simulink model "FOC"  (Simulink 7.5)
settings: Solver=ode3  StartTime=0.0  StopTime=1  FixedStep=1e-5  RelTol=1e-3
libraries: powerlib x5, simulink x1
settings Model: Creator=lenovo  LastModifiedBy=Administrator

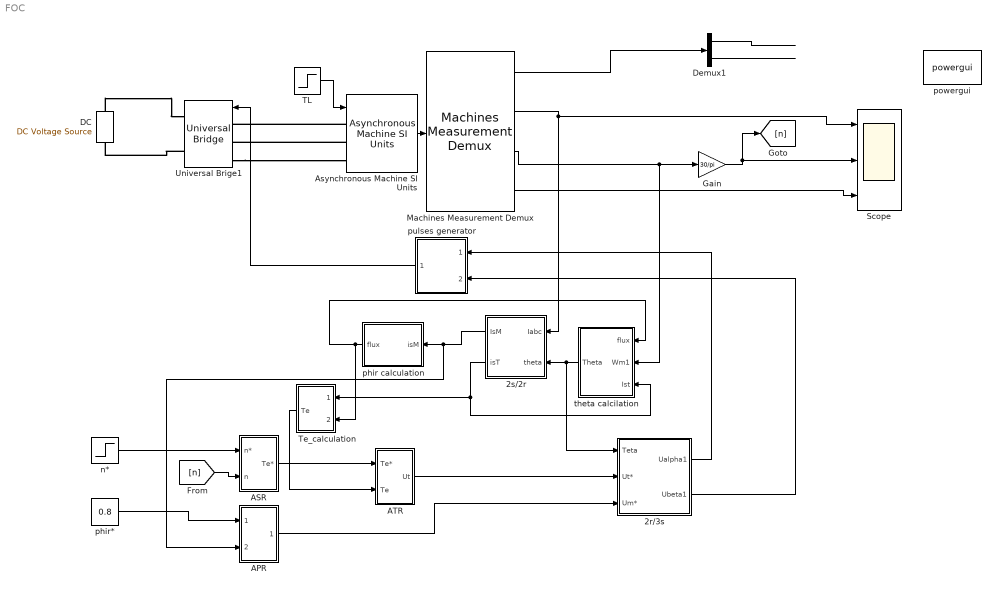
== system FOC ==
  2r/3s : Subsystem
  2s/2r : Subsystem
  APR : Subsystem
  ASR : Subsystem
  ATR : Subsystem
  Asynchronous Machine SI Units : powerlib/Machines/Asynchronous Machine SI Units  DialogController=POWERSYS.PowerSysDialog  SystemSampleTime=-1  PresetModel="17:  20 HP (15KW)   400 V 50Hz 1460 RPM"  MechanicalLoad=Torque Tm  ShowDetailedParameters=on  RotorType=Squirrel-cage  ReferenceFrame=Stationary  NominalParameters=[1.5e+004 400 50]  Stator=[0.2147 0.000991]  Rotor=[0.2205 0.000991]  Lm=0.06419  Mechanical=[0.102 0.009541 2]  PolePairs=2  InitialConditions="[ 1,0   0,0,0   0,0,0 ]"  Units=SI  LoadFlowParameters=0  SimulateSaturation=off  Saturation=[9.9249,19.6672,38.0377,51.3988,69.2824,105.1337,152.5532,214.2421,303.1917;230, 322, 414, 460, 506, 552, 598, 644, 690]  TsPowergui=0  TsBlock=-1  IterativeModel=Forward Euler
  "DC " : powerlib/Electrical Sources/DC Voltage Source  DialogController=POWERSYS.PowerSysDialog  SystemSampleTime=-1  Amplitude=650  Measurements=None
  Demux1 : Demux  Outputs=2
  Gain : Gain  Gain=30/pi
  Machines Measurement Demux : powerlib/Machines/Machines Measurement Demux  DialogController=POWERSYS.PowerSysDialog  SystemSampleTime=-1  machType=Asynchronous  ssm1=on  ssm2=on  ssm3=on  ssm4=on  ssm5=on  ssm6=on  sm1=off  sm2=off  sm3=off  sm4=off  sm5=off  sm6=off  sm7=off  sm8=on  sm9=off  sm10=off  sm11=off  sm115=off  sm12=off  sm13=off  sm14=off  asm1=off  asm2=off  asm3=on  asm4=off  asm5=on  asm6=off  asm7=off  asm8=off  asm9=on  asm10=on  asm11=off  pmsm1=on  pmsm2=on  pmsm3=on  pmsm4=off  pmsm5=on  pmsm6=on  pmsm7=on  lastType=1
  Scope : Scope  NumInputPorts=3
      settings: YMin=-400~0~-250  YMax=450~1500~350  SaveName=ScopeData3
  TL : Step  Time=0.4  After=0  SampleTime=0
  Te_calculation : Subsystem
  Universal Brige1 : powerlib/Power Electronics/Universal Bridge  DialogController=POWERSYS.PowerSysDialog  SystemSampleTime=-1  Arms=3  SnubberResistance=1e5  SnubberCapacitance=inf  Device=IGBT / Diodes  Ron=1e-3  Lon=0  ForwardVoltages="[  0  0  ]"  ForwardVoltage=0  GTOparameters=[ 10e-6 , 20e-6 ]  IGBTparameters=[ 1e-6 , 2e-6 ]  Measurements=All voltages and currents  Measurements_2=None  converterType=Rectifier
  n* : Step  Time=0.5  Before=1420  After=1200  SampleTime=0
  phir calculation : Subsystem
  phir* : Constant  Value=0.8
  powergui : powerlib/powergui  Priority=1  SystemSampleTime=-1  SimulationMode=Continuous  SampleTime=50e-6  frequency=60  SPID=off  DisableSnubberDevices=off  DisableRonSwitches=off  DisableVfSwitches=off  SwTol=0  Interpol=off  frequencyindice=50  echomessages=off  HookPort=off  DisplayEquations=off  FunctionMessages=off  EnableUseOfTLC=off  x0status=blocks  RestoreLinks=warning  ResistiveCurrentMeasurement=off  Ylog=off  Xlog=on  ShowGrid=off  save=off  variable=ZData  ZoomFFT=off  StartTime=0.0  cycles=1  DisplayStyle=1  FreqAxis=off  MaxFrequency=1000  frequencyindicesteady=1  display=off  methode=off
  pulses generator : Subsystem
  theta calcilation : Subsystem
  wires:
  TL/1 -> Asynchronous Machine SI Units/1
  phir calculation/1(flux) -> Te_calculation/2(flux), theta calcilation/1(flux)
  n*/1 -> ASR/1(n*)
  ATR/1(Ut) -> 2r/3s/2(Ut*)
  phir*/1 -> APR/1(phir*)
  APR/1(Um) -> 2r/3s/3(Um*)
  Asynchronous Machine SI Units/1 -> Machines Measurement Demux/1
  Machines Measurement Demux/2 -> Scope/1, 2s/2r/1(Iabc)
  Machines Measurement Demux/3 -> Gain/1, theta calcilation/2(Wm1)
  Gain/1 -> [n], Scope/2
  [n] -> ASR/2(n)
  Machines Measurement Demux/4 -> Scope/3
  2s/2r/1(IsM) -> phir calculation/1(isM), APR/2(phir)
  theta calcilation/1(Theta) -> 2s/2r/2(theta), 2r/3s/1(Teta)
  2s/2r/2(isT) -> theta calcilation/3(Ist), Te_calculation/1(i_sT)
  Machines Measurement Demux/1 -> Demux1/1
  ASR/1(Te*) -> ATR/1(Te*)
  pulses generator/1(SVPWM) -> Universal Brige1/1
  2r/3s/1(Ualpha1) -> pulses generator/1(Ualpha)
  2r/3s/2(Ubeta1) -> pulses generator/2(Ubeta)
  Demux1/1 -> ?
  Demux1/2 -> ?
  Te_calculation/1(Te) -> ATR/2(Te)
  connections:
  "DC "/RConn1 -- Universal Brige1/RConn1
  Universal Brige1/RConn2 -- "DC "/LConn1
  Asynchronous Machine SI Units/LConn1 -- Universal Brige1/LConn1
  Asynchronous Machine SI Units/LConn2 -- Universal Brige1/LConn2
  Universal Brige1/LConn3 -- Asynchronous Machine SI Units/LConn3

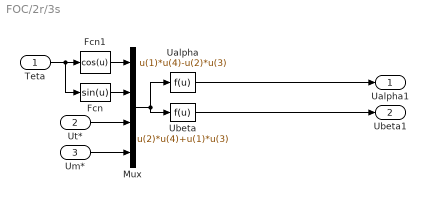
== system FOC/2r/3s ==
  Teta : Inport
  Ut* : Inport  Port=2
  Um* : Inport  Port=3
  Fcn : Fcn  Expr=sin(u)
  Fcn1 : Fcn  Expr=cos(u)
  Mux : Mux
  Ualpha : Fcn  Expr=u(1)*u(4)-u(2)*u(3)
  Ubeta : Fcn  Expr=u(2)*u(4)+u(1)*u(3)
  Ualpha1 : Outport  InitialOutput=0
  Ubeta1 : Outport  Port=2  InitialOutput=0
  wires:
  Um*/1 -> Mux/4
  Ut*/1 -> Mux/3
  Teta/1 -> Fcn/1, Fcn1/1
  Mux/1 -> Ualpha/1, Ubeta/1
  Fcn1/1 -> Mux/1
  Fcn/1 -> Mux/2
  Ualpha/1 -> Ualpha1/1
  Ubeta/1 -> Ubeta1/1

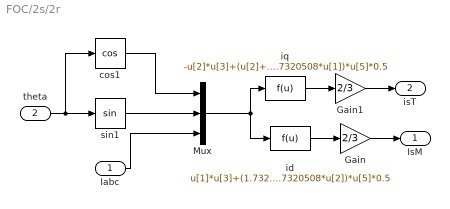
== system FOC/2s/2r ==
  Iabc : Inport
  theta : Inport  Port=2
  Gain : Gain  Gain=2/3  SaturateOnIntegerOverflow=on  OutDataTypeStr=Inherit: Same as input  ParamDataTypeStr=Inherit: Same as input
  Gain1 : Gain  Gain=2/3  SaturateOnIntegerOverflow=on  OutDataTypeStr=Inherit: Same as input  ParamDataTypeStr=Inherit: Same as input
  Mux : Mux  Inputs=3
  cos1 : Trigonometry  Operator=cos
  id : Fcn  Expr=u[1]*u[3]+(1.7320508*u[2]-u[1])*u[4]*0.5+(-u[1]-1.7320508*u[2])*u[5]*0.5
  iq : Fcn  Expr=-u[2]*u[3]+(u[2]+1.7320508*u[1])*u[4]*0.5+(u[2]-1.7320508*u[1])*u[5]*0.5
  sin1 : Trigonometry
  IsM : Outport  InitialOutput=0
  isT : Outport  Port=2  InitialOutput=0
  wires:
  Iabc/1 -> Mux/3
  iq/1 -> Gain1/1
  id/1 -> Gain/1
  Gain/1 -> IsM/1
  Gain1/1 -> isT/1
  Mux/1 -> iq/1, id/1
  cos1/1 -> Mux/1
  sin1/1 -> Mux/2
  theta/1 -> sin1/1, cos1/1

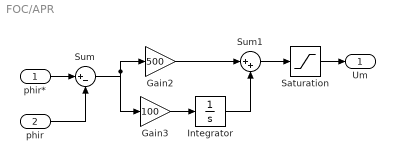
== system FOC/APR ==
  phir* : Inport
  phir : Inport  Port=2
  Gain2 : Gain  Gain=500
  Gain3 : Gain  Gain=100
  Integrator : Integrator  LimitOutput=on  UpperSaturationLimit=13  LowerSaturationLimit=-13
  Saturation : Saturate  UpperLimit=500  LowerLimit=-500
  Sum : Sum  Inputs=|+-
  Sum1 : Sum  Inputs=|++
  Um : Outport
  wires:
  Sum/1 -> Gain2/1, Gain3/1
  Gain2/1 -> Sum1/1
  Gain3/1 -> Integrator/1
  Integrator/1 -> Sum1/2
  Sum1/1 -> Saturation/1
  Saturation/1 -> Um/1
  phir*/1 -> Sum/1
  phir/1 -> Sum/2

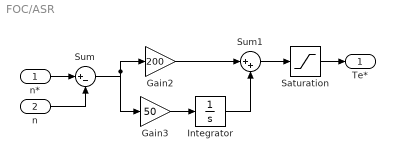
== system FOC/ASR ==
  n* : Inport
  n : Inport  Port=2
  Gain2 : Gain  Gain=200
  Gain3 : Gain  Gain=50
  Integrator : Integrator  LimitOutput=on  UpperSaturationLimit=200  LowerSaturationLimit=-200
  Saturation : Saturate  UpperLimit=200  LowerLimit=-200
  Sum : Sum  Inputs=|+-
  Sum1 : Sum  Inputs=|++
  Te* : Outport
  wires:
  Sum/1 -> Gain2/1, Gain3/1
  Gain2/1 -> Sum1/1
  Gain3/1 -> Integrator/1
  Integrator/1 -> Sum1/2
  Sum1/1 -> Saturation/1
  Saturation/1 -> Te*/1
  n*/1 -> Sum/1
  n/1 -> Sum/2

== system FOC/ATR ==
  Te* : Inport
  Te : Inport  Port=2
  Gain2 : Gain  Gain=500
  Gain3 : Gain  Gain=50
  Integrator : Integrator  LimitOutput=on  UpperSaturationLimit=200  LowerSaturationLimit=-80
  Saturation : Saturate  UpperLimit=500  LowerLimit=-500
  Sum : Sum  Inputs=|+-
  Sum1 : Sum  Inputs=|++
  Ut : Outport
  wires:
  Sum/1 -> Gain2/1, Gain3/1
  Gain2/1 -> Sum1/1
  Gain3/1 -> Integrator/1
  Integrator/1 -> Sum1/2
  Sum1/1 -> Saturation/1
  Saturation/1 -> Ut/1
  Te*/1 -> Sum/1
  Te/1 -> Sum/2

== system FOC/Te_calculation ==
  i_sT : Inport  OutDataType=fixdt(1, 16)  OutScaling=2^0
  flux : Inport  Port=2  OutDataType=fixdt(1, 16)  OutScaling=2^0
  Gain : Gain  Gain=1/0.50771927  ParameterDataType=fixdt(1, 16)  ParameterScaling=2^0  OutDataType=fixdt(1, 16)  OutScaling=2^0
  Product : Product  OutDataType=fixdt(1, 16)  OutScaling=2^0  RndMeth=Zero
  Te : Outport  OutDataType=fixdt(1, 16)  OutScaling=2^0
  wires:
  flux/1 -> Product/2
  i_sT/1 -> Gain/1
  Product/1 -> Te/1
  Gain/1 -> Product/1

== system FOC/phir calculation ==
  isM : Inport
  Transfer Fcn : TransferFcn  Numerator=[0.06419]  Denominator=[0.2956 1]
  flux : Outport
  wires:
  isM/1 -> Transfer Fcn/1
  Transfer Fcn/1 -> flux/1

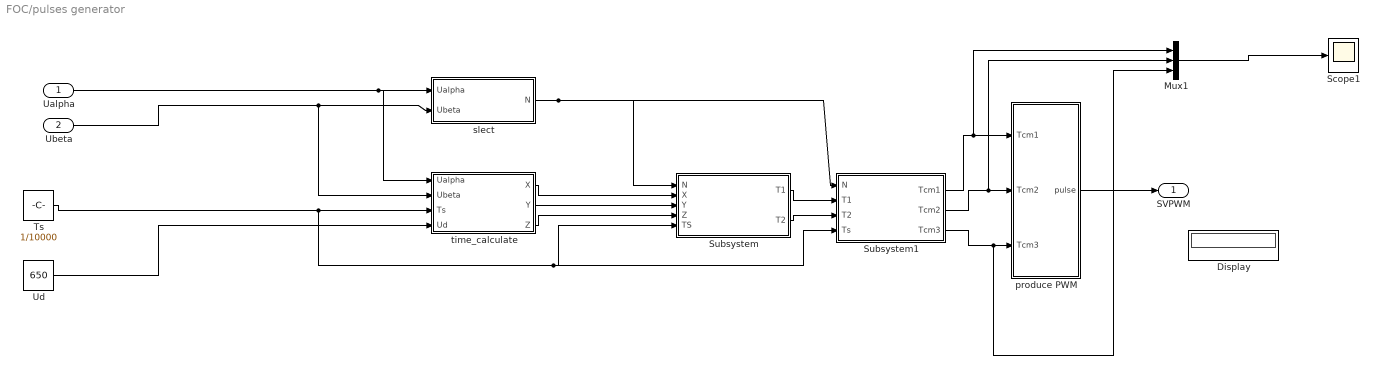
== system FOC/pulses generator ==
  Ualpha : Inport  OutDataType=fixdt(1, 16)  OutScaling=2^0
  Ubeta : Inport  Port=2  OutDataType=fixdt(1, 16)  OutScaling=2^0
  Display : Display
  Mux1 : Mux  Inputs=3
  Scope1 : Scope
      settings: TimeRange=0.2  YMin=3.5e-005  YMax=6.5e-005  SaveName=ScopeData2
  Subsystem : Subsystem
  Subsystem1 : Subsystem
  Ts : Constant  Value=1/10000  OutDataType=fixdt(1, 16)  OutScaling=2^0
  Ud : Constant  Value=650  OutDataType=fixdt(1, 16)  OutScaling=2^0
  produce PWM : Subsystem
  slect : Subsystem
  time_calculate : Subsystem
  SVPWM : Outport  OutDataType=fixdt(1, 16)  OutScaling=2^0
  wires:
  Ualpha/1 -> time_calculate/1(Ualpha), slect/1(Ualpha)
  slect/1(N) -> Subsystem/1(N), Subsystem1/1(N)
  Subsystem/1(T1) -> Subsystem1/2(T1)
  Subsystem/2(T2) -> Subsystem1/3(T2)
  Subsystem1/1(Tcm1) -> produce PWM/1(Tcm1), Mux1/1
  Ts/1 -> time_calculate/3(Ts), Subsystem/5(TS), Subsystem1/4(Ts)
  Ud/1 -> time_calculate/4(Ud)
  Subsystem1/2(Tcm2) -> produce PWM/2(Tcm2), Mux1/2
  Subsystem1/3(Tcm3) -> produce PWM/3(Tcm3), Mux1/3
  time_calculate/1(X) -> Subsystem/2(X)
  time_calculate/2(Y) -> Subsystem/3(Y)
  time_calculate/3(Z) -> Subsystem/4(Z)
  Mux1/1 -> Scope1/1
  Ubeta/1 -> slect/2(Ubeta), time_calculate/2(Ubeta)
  produce PWM/1(pulse) -> SVPWM/1

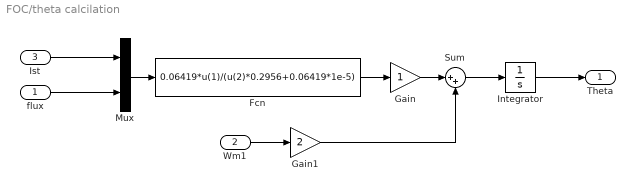
== system FOC/theta calcilation ==
  flux : Inport
  Wm1 : Inport  Port=2
  Ist : Inport  Port=3
  Fcn : Fcn  Expr=0.06419*u(1)/(u(2)*0.2956+0.06419*1e-5)
  Gain : Gain
  Gain1 : Gain  Gain=2
  Integrator : Integrator  InitialCondition=1e-6  LimitOutput=on  UpperSaturationLimit=1e6  LowerSaturationLimit=-1e6
  Mux : Mux  Inputs=2
  Sum : Sum  Inputs=|++
  Theta : Outport
  wires:
  Ist/1 -> Mux/1
  flux/1 -> Mux/2
  Mux/1 -> Fcn/1
  Fcn/1 -> Gain/1
  Gain/1 -> Sum/1
  Gain1/1 -> Sum/2
  Sum/1 -> Integrator/1
  Integrator/1 -> Theta/1
  Wm1/1 -> Gain1/1

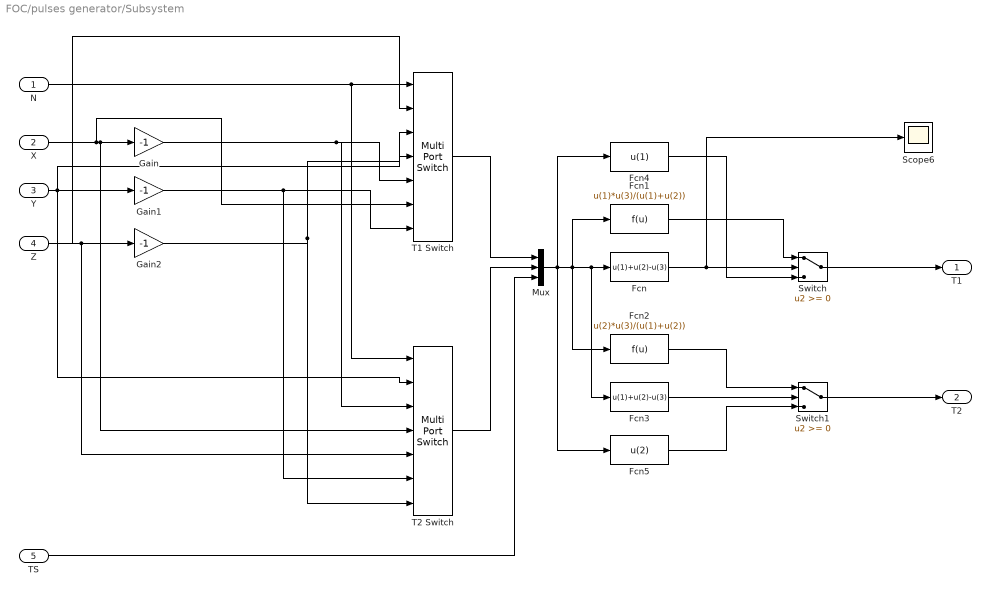
== system FOC/pulses generator/Subsystem ==
  N : Inport  OutDataType=fixdt(1, 16)  OutScaling=2^0
  X : Inport  Port=2  OutDataType=fixdt(1, 16)  OutScaling=2^0
  Y : Inport  Port=3  OutDataType=fixdt(1, 16)  OutScaling=2^0
  Z : Inport  Port=4  OutDataType=fixdt(1, 16)  OutScaling=2^0
  TS : Inport  Port=5  OutDataType=fixdt(1, 16)  OutScaling=2^0
  Fcn : Fcn  Expr=u(1)+u(2)-u(3)
  Fcn1 : Fcn  Expr=u(1)*u(3)/(u(1)+u(2))
  Fcn2 : Fcn  Expr=u(2)*u(3)/(u(1)+u(2))
  Fcn3 : Fcn  Expr=u(1)+u(2)-u(3)
  Fcn4 : Fcn  Expr=u(1)
  Fcn5 : Fcn  Expr=u(2)
  Gain : Gain  Gain=-1  ParameterDataType=fixdt(1, 16)  ParameterScaling=2^0  OutDataType=fixdt(1, 16)  OutScaling=2^0
  Gain1 : Gain  Gain=-1  ParameterDataType=fixdt(1, 16)  ParameterScaling=2^0  OutDataType=fixdt(1, 16)  OutScaling=2^0
  Gain2 : Gain  Gain=-1  ParameterDataType=fixdt(1, 16)  ParameterScaling=2^0  OutDataType=fixdt(1, 16)  OutScaling=2^0
  Mux : Mux  Inputs=3
  Scope6 : Scope
      settings: TimeRange=0.2  YMin=-1.05e-005  YMax=-4e-006  SaveName=ScopeData5  SampleTime=0.000001
  Switch : Switch  OutDataType=fixdt(1, 16)  OutScaling=2^0
  Switch1 : Switch  OutDataType=fixdt(1, 16)  OutScaling=2^0
  T1 Switch : MultiPortSwitch  Inputs=6  zeroidx=off  OutDataType=fixdt(1, 16)  OutScaling=2^0
  T2 Switch : MultiPortSwitch  Inputs=6  zeroidx=off  OutDataType=fixdt(1, 16)  OutScaling=2^0
  T1 : Outport  OutDataType=fixdt(1, 16)  OutScaling=2^0
  T2 : Outport  Port=2  OutDataType=fixdt(1, 16)  OutScaling=2^0
  wires:
  N/1 -> T1 Switch/1, T2 Switch/1
  X/1 -> Gain/1, T2 Switch/4, T1 Switch/6
  Y/1 -> Gain1/1, T2 Switch/2, T1 Switch/3
  Z/1 -> Gain2/1, T1 Switch/2, T2 Switch/5
  Gain/1 -> T2 Switch/3, T1 Switch/5
  Gain2/1 -> T1 Switch/4, T2 Switch/7
  Gain1/1 -> T2 Switch/6, T1 Switch/7
  T1 Switch/1 -> Mux/1
  T2 Switch/1 -> Mux/2
  TS/1 -> Mux/3
  Mux/1 -> Fcn1/1, Fcn/1, Fcn3/1, Fcn2/1, Fcn4/1, Fcn5/1
  Fcn3/1 -> Switch1/2
  Switch/1 -> T1/1
  Switch1/1 -> T2/1
  Fcn4/1 -> Switch/3
  Fcn/1 -> Switch/2, Scope6/1
  Fcn1/1 -> Switch/1
  Fcn2/1 -> Switch1/1
  Fcn5/1 -> Switch1/3

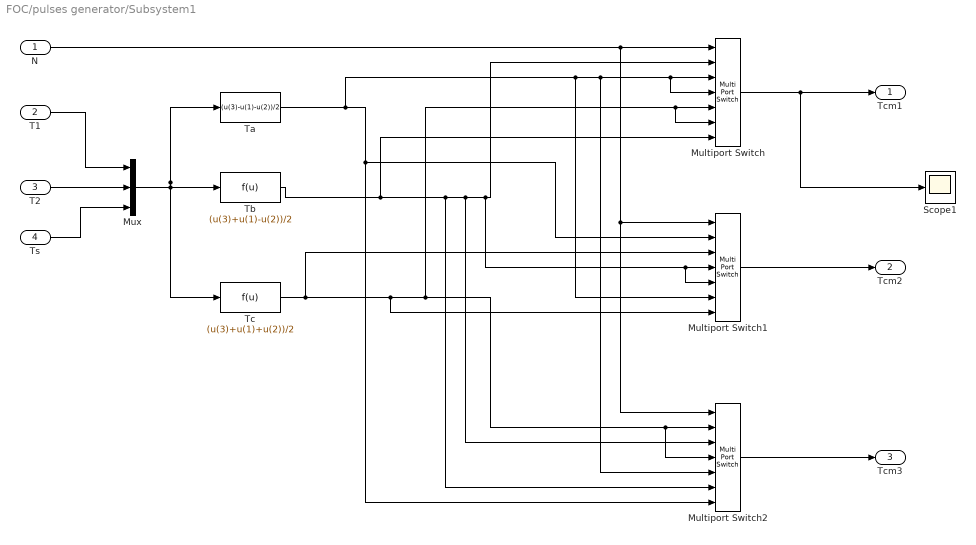
== system FOC/pulses generator/Subsystem1 ==
  N : Inport  OutDataType=fixdt(1, 16)  OutScaling=2^0
  T1 : Inport  Port=2  OutDataType=fixdt(1, 16)  OutScaling=2^0
  T2 : Inport  Port=3  OutDataType=fixdt(1, 16)  OutScaling=2^0
  Ts : Inport  Port=4  OutDataType=fixdt(1, 16)  OutScaling=2^0
  Multiport Switch : MultiPortSwitch  Inputs=6  zeroidx=off  OutDataType=fixdt(1, 16)  OutScaling=2^0
  Multiport Switch1 : MultiPortSwitch  Inputs=6  zeroidx=off  OutDataType=fixdt(1, 16)  OutScaling=2^0
  Multiport Switch2 : MultiPortSwitch  Inputs=6  zeroidx=off  OutDataType=fixdt(1, 16)  OutScaling=2^0
  Mux : Mux  Inputs=3
  Scope1 : Scope
      settings: YMin=-2.5e-006  YMax=2.75e-005  SaveName=ScopeData4
  Ta : Fcn  Expr=(u(3)-u(1)-u(2))/2
  Tb : Fcn  Expr=(u(3)+u(1)-u(2))/2
  Tc : Fcn  Expr=(u(3)+u(1)+u(2))/2
  Tcm1 : Outport  OutDataType=fixdt(1, 16)  OutScaling=2^0
  Tcm2 : Outport  Port=2  OutDataType=fixdt(1, 16)  OutScaling=2^0
  Tcm3 : Outport  Port=3  OutDataType=fixdt(1, 16)  OutScaling=2^0
  wires:
  Ts/1 -> Mux/3
  Multiport Switch/1 -> Tcm1/1, Scope1/1
  Multiport Switch1/1 -> Tcm2/1
  Multiport Switch2/1 -> Tcm3/1
  T1/1 -> Mux/1
  N/1 -> Multiport Switch/1, Multiport Switch1/1, Multiport Switch2/1
  T2/1 -> Mux/2
  Tb/1 -> Multiport Switch/2, Multiport Switch1/4, Multiport Switch1/5, Multiport Switch2/3, Multiport Switch2/6, Multiport Switch/7
  Ta/1 -> Multiport Switch1/2, Multiport Switch2/7, Multiport Switch1/6, Multiport Switch/3, Multiport Switch/4, Multiport Switch2/5
  Tc/1 -> Multiport Switch1/3, Multiport Switch2/2, Multiport Switch2/4, Multiport Switch/5, Multiport Switch/6, Multiport Switch1/7
  Mux/1 -> Tb/1, Ta/1, Tc/1

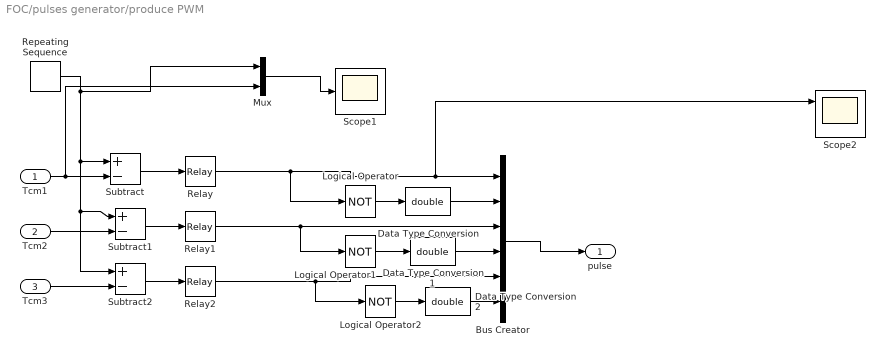
== system FOC/pulses generator/produce PWM ==
  Tcm1 : Inport
  Tcm2 : Inport  Port=2
  Tcm3 : Inport  Port=3
  Bus Creator : BusCreator  Inputs=6
  Data Type Conversion : DataTypeConversion  OutDataTypeMode=double  OutDataTypeStr=double
  Data Type Conversion1 : DataTypeConversion  OutDataTypeMode=double  OutDataTypeStr=double
  Data Type Conversion2 : DataTypeConversion  OutDataTypeMode=double  OutDataTypeStr=double
  Logical Operator : Logic  Operator=NOT  AllPortsSameDT=off
  Logical Operator1 : Logic  Operator=NOT  AllPortsSameDT=off
  Logical Operator2 : Logic  Operator=NOT  AllPortsSameDT=off
  Mux : Mux  Inputs=2
  Relay : Relay
  Relay1 : Relay
  Relay2 : Relay
  Repeating Sequence : simulink/Sources/Repeating Sequence  SystemSampleTime=-1  rep_seq_t=[0 1/10000 2/10000]  rep_seq_y=[0 1/10000 0]
  Scope1 : Scope
      settings: TimeRange=0.1  YMin=0  YMax=0.000105
  Scope2 : Scope  NumInputPorts=2
      settings: TimeRange=0.01  YMin=0~-1  YMax=1~1
  Subtract : Sum  Inputs=+-
  Subtract1 : Sum  Inputs=+-
  Subtract2 : Sum  Inputs=+-
  pulse : Outport
  wires:
  Subtract/1 -> Relay/1
  Subtract1/1 -> Relay1/1
  Subtract2/1 -> Relay2/1
  Repeating Sequence/1 -> Subtract/1, Subtract2/1, Subtract1/1, Mux/1
  Tcm1/1 -> Subtract/2, Mux/2
  Tcm2/1 -> Subtract1/2
  Tcm3/1 -> Subtract2/2
  Logical Operator1/1 -> Data Type Conversion1/1
  Logical Operator2/1 -> Data Type Conversion2/1
  Logical Operator/1 -> Data Type Conversion/1
  Relay/1 -> Logical Operator/1, Bus Creator/1, Scope2/1
  Relay1/1 -> Bus Creator/3, Logical Operator1/1
  Relay2/1 -> Bus Creator/5, Logical Operator2/1
  Bus Creator/1 -> pulse/1
  Data Type Conversion/1 -> Bus Creator/2
  Data Type Conversion1/1 -> Bus Creator/4
  Data Type Conversion2/1 -> Bus Creator/6
  Mux/1 -> Scope1/1

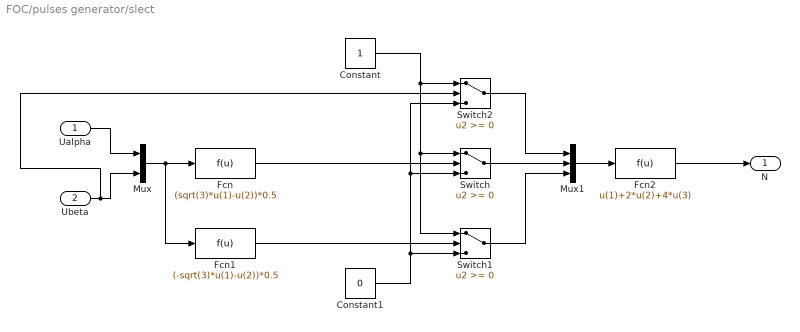
== system FOC/pulses generator/slect ==
  Ualpha : Inport  OutDataType=fixdt(1, 16)  OutScaling=2^0
  Ubeta : Inport  Port=2  OutDataType=fixdt(1, 16)  OutScaling=2^0
  Constant : Constant  OutDataType=fixdt(1, 16)  OutScaling=2^0
  Constant1 : Constant  Value=0  OutDataType=fixdt(1, 16)  OutScaling=2^0
  Fcn : Fcn  Expr=(sqrt(3)*u(1)-u(2))*0.5
  Fcn1 : Fcn  Expr=(-sqrt(3)*u(1)-u(2))*0.5
  Fcn2 : Fcn  Expr=u(1)+2*u(2)+4*u(3)
  Mux : Mux  Inputs=2
  Mux1 : Mux  Inputs=3
  Switch : Switch  OutDataType=fixdt(1, 16)  OutScaling=2^0
  Switch1 : Switch  OutDataType=fixdt(1, 16)  OutScaling=2^0
  Switch2 : Switch  OutDataType=fixdt(1, 16)  OutScaling=2^0
  N : Outport  OutDataType=fixdt(1, 16)  OutScaling=2^0
  wires:
  Ualpha/1 -> Mux/1
  Ubeta/1 -> Mux/2, Switch2/2
  Mux/1 -> Fcn/1, Fcn1/1
  Fcn1/1 -> Switch1/2
  Fcn/1 -> Switch/2
  Constant/1 -> Switch2/1, Switch/1, Switch1/1
  Constant1/1 -> Switch1/3, Switch/3, Switch2/3
  Switch2/1 -> Mux1/1
  Switch/1 -> Mux1/2
  Switch1/1 -> Mux1/3
  Mux1/1 -> Fcn2/1
  Fcn2/1 -> N/1

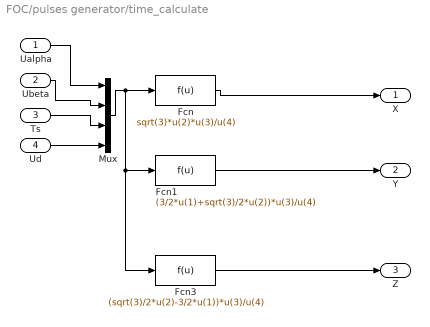
== system FOC/pulses generator/time_calculate ==
  Ualpha : Inport  OutDataType=fixdt(1, 16)  OutScaling=2^0
  Ubeta : Inport  Port=2  OutDataType=fixdt(1, 16)  OutScaling=2^0
  Ts : Inport  Port=3  OutDataType=fixdt(1, 16)  OutScaling=2^0
  Ud : Inport  Port=4  OutDataType=fixdt(1, 16)  OutScaling=2^0
  Fcn : Fcn  Expr=sqrt(3)*u(2)*u(3)/u(4)
  Fcn1 : Fcn  Expr=(3/2*u(1)+sqrt(3)/2*u(2))*u(3)/u(4)
  Fcn3 : Fcn  Expr=(sqrt(3)/2*u(2)-3/2*u(1))*u(3)/u(4)
  Mux : Mux
  X : Outport  OutDataType=fixdt(1, 16)  OutScaling=2^0
  Y : Outport  Port=2  OutDataType=fixdt(1, 16)  OutScaling=2^0
  Z : Outport  Port=3  OutDataType=fixdt(1, 16)  OutScaling=2^0
  wires:
  Ualpha/1 -> Mux/1
  Ubeta/1 -> Mux/2
  Mux/1 -> Fcn/1, Fcn1/1, Fcn3/1
  Ts/1 -> Mux/3
  Ud/1 -> Mux/4
  Fcn/1 -> X/1
  Fcn1/1 -> Y/1
  Fcn3/1 -> Z/1
